simulink model "EHP_test"  (Simulink 7.4)
settings: Solver=FixedStepDiscrete  StartTime=0.0  StopTime=inf  FixedStep=0.01  RelTol=1e-3
undefined symbols (not defined in the file): EHPc_BatIsoTestCmd, EHPc_r_ClcnRo, EHPc_r_IsoDiag_limit, EHPc_r_IsoDiagInitVal, EHPc_r_IsoDiagWarn_limit
libraries: simulink x5
settings Model: Creator=zhaoxiangri  LastModifiedBy=sunsijun

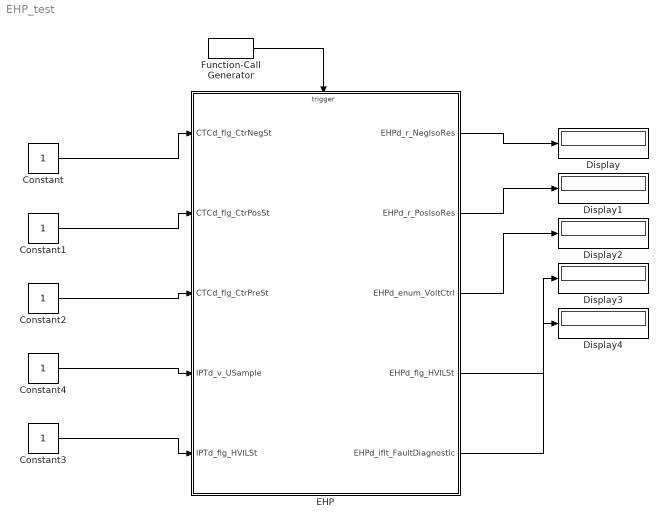
== system EHP_test ==
  Constant{,1..3} (4 alike) : Constant  OutDataTypeMode=boolean  OutDataType=fixdt(1, 16)  OutScaling=2^0  OutDataTypeStr=boolean
  Constant4 : Constant  OutDataTypeMode=single  OutDataType=fixdt(1, 16)  OutScaling=2^0  OutDataTypeStr=single
  Display{,1..4} (5 alike) : Display
  EHP : Subsystem  TreatAsAtomicUnit=on
  Function-Call Generator : simulink/Ports & Subsystems/Function-Call Generator  sample_time=1  numberOfIterations=1
  wires:
  Function-Call Generator/1 -> EHP/Trigger
  Constant/1 -> EHP/1(CTCd_flg_CtrNegSt)
  Constant1/1 -> EHP/2(CTCd_flg_CtrPosSt)
  Constant2/1 -> EHP/3(CTCd_flg_CtrPreSt)
  Constant3/1 -> EHP/5(IPTd_flg_HVILSt)
  Constant4/1 -> EHP/4(IPTd_v_USample)
  EHP/1(EHPd_r_NegIsoRes) -> Display/1
  EHP/2(EHPd_r_PosIsoRes) -> Display1/1
  EHP/3(EHPd_enum_VoltCtrl) -> Display2/1
  EHP/4(EHPd_flg_HVILSt) -> Display3/1
  EHP/5(EHPd_iflt_FaultDiagnostic) -> Display4/1

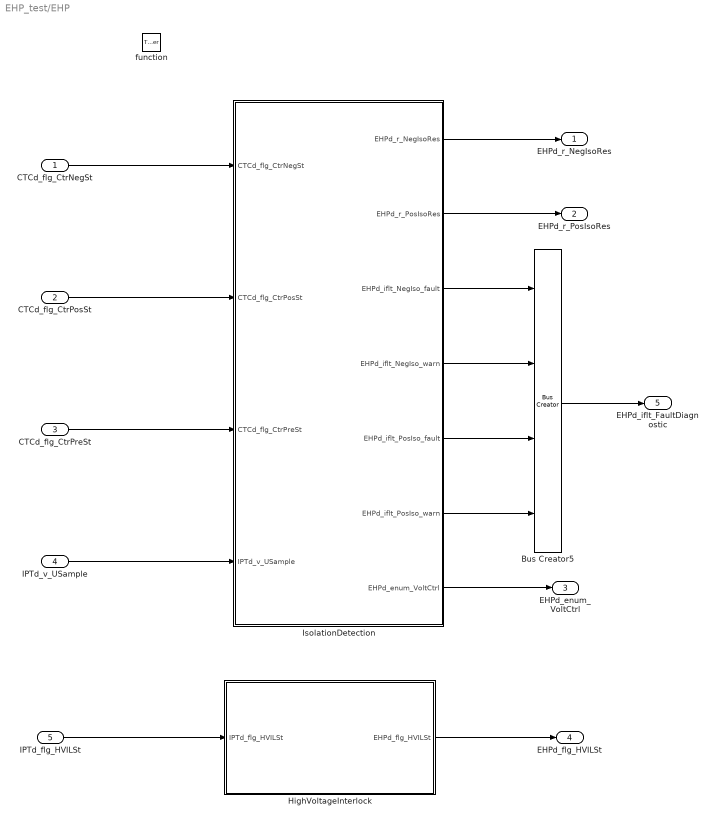
== system EHP_test/EHP ==
  CTCd_flg_CtrNegSt : Inport  OutDataType=fixdt(1, 16)  OutScaling=2^0
  CTCd_flg_CtrPosSt : Inport  Port=2  OutDataType=fixdt(1, 16)  OutScaling=2^0
  CTCd_flg_CtrPreSt : Inport  Port=3  OutDataType=fixdt(1, 16)  OutScaling=2^0
  IPTd_v_USample : Inport  Port=4  OutDataType=fixdt(1, 16)  OutScaling=2^0
  IPTd_flg_HVILSt : Inport  Port=5  OutDataType=fixdt(1, 16)  OutScaling=2^0
  function : TriggerPort  TriggerType=function-call
  Bus Creator5 : BusCreator
  HighVoltageInterlock : Subsystem  RTWFcnName=HighVoltageInterlock
      settings: RTWSystemCode=Function  RTWFcnNameOpts=User specified  RTWFileNameOpts=Use function name
  IsolationDetection : Subsystem  Description=|
      | $Author:Yan LiJuan$
      | $Date:2015/03/26$  
      | $Revision:1.0$
  EHPd_r_NegIsoRes : Outport  OutDataType=fixdt(1, 16)  OutScaling=2^0
  EHPd_r_PosIsoRes : Outport  Port=2  OutDataType=fixdt(1, 16)  OutScaling=2^0
  EHPd_enum_VoltCtrl : Outport  Port=3  OutDataType=fixdt(1, 16)  OutScaling=2^0
  EHPd_flg_HVILSt : Outport  Port=4  OutDataType=fixdt(1, 16)  OutScaling=2^0
  EHPd_iflt_FaultDiagnostic : Outport  Port=5  OutDataType=fixdt(1, 16)  OutScaling=2^0
  wires:
  IsolationDetection/7(EHPd_enum_VoltCtrl) -> EHPd_enum_VoltCtrl/1
  IsolationDetection/2(EHPd_r_PosIsoRes) -> EHPd_r_PosIsoRes/1
  IsolationDetection/1(EHPd_r_NegIsoRes) -> EHPd_r_NegIsoRes/1
  IPTd_flg_HVILSt/1 -> HighVoltageInterlock/1(IPTd_flg_HVILSt)
  HighVoltageInterlock/1(EHPd_flg_HVILSt) -> EHPd_flg_HVILSt/1
  IPTd_v_USample/1 -> IsolationDetection/4(IPTd_v_USample)
  CTCd_flg_CtrPreSt/1 -> IsolationDetection/3(CTCd_flg_CtrPreSt)
  CTCd_flg_CtrPosSt/1 -> IsolationDetection/2(CTCd_flg_CtrPosSt)
  CTCd_flg_CtrNegSt/1 -> IsolationDetection/1(CTCd_flg_CtrNegSt)
  IsolationDetection/3(EHPd_iflt_NegIso_fault) -> Bus Creator5/1
  IsolationDetection/4(EHPd_iflt_NegIso_warn) -> Bus Creator5/2
  IsolationDetection/5(EHPd_iflt_PosIso_fault) -> Bus Creator5/3
  IsolationDetection/6(EHPd_iflt_PosIso_warn) -> Bus Creator5/4
  Bus Creator5/1 -> EHPd_iflt_FaultDiagnostic/1

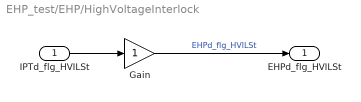
== system EHP_test/EHP/HighVoltageInterlock ==
  IPTd_flg_HVILSt : Inport  OutDataType=fixdt(1, 16)  OutScaling=2^0
  Gain : Gain  ParameterDataType=fixdt(1, 16)  ParameterScaling=2^0  OutDataType=fixdt(1, 16)  OutScaling=2^0
  EHPd_flg_HVILSt : Outport  OutDataType=fixdt(1, 16)  OutScaling=2^0
  wires:
  IPTd_flg_HVILSt/1 -> Gain/1
  Gain/1 -> EHPd_flg_HVILSt/1  "EHPd_flg_HVILSt"

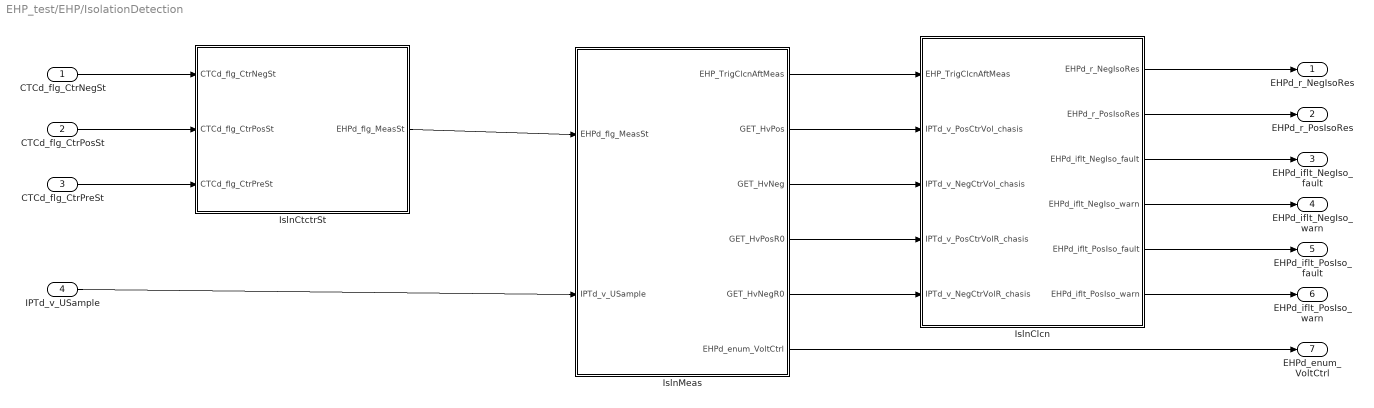
== system EHP_test/EHP/IsolationDetection ==
  CTCd_flg_CtrNegSt : Inport  OutDataType=fixdt(1, 16)  OutScaling=2^0
  CTCd_flg_CtrPosSt : Inport  Port=2  OutDataType=fixdt(1, 16)  OutScaling=2^0
  CTCd_flg_CtrPreSt : Inport  Port=3  OutDataType=fixdt(1, 16)  OutScaling=2^0
  IPTd_v_USample : Inport  Port=4  OutDataType=fixdt(1, 16)  OutScaling=2^0
  IslnClcn : Subsystem  Description=|
      | $Author:Yan LiJuan$
      | $Date:2015/03/26$  
      | $Revision:1.0$
  IslnCtctrSt : Subsystem  Description=|
      | $Author:Yan LiJuan$
      | $Date:2015/03/26$  
      | $Revision:1.0$
  IslnMeas : Subsystem  Description=|
      | $Author:Yan LiJuan$
      | $Date:2015/03/26$  
      | $Revision:1.0$
  EHPd_r_NegIsoRes : Outport  OutDataType=fixdt(1, 16)  OutScaling=2^0
  EHPd_r_PosIsoRes : Outport  Port=2  OutDataType=fixdt(1, 16)  OutScaling=2^0
  EHPd_iflt_NegIso_fault : Outport  Port=3  OutDataType=fixdt(1, 16)  OutScaling=2^0
  EHPd_iflt_NegIso_warn : Outport  Port=4  OutDataType=fixdt(1, 16)  OutScaling=2^0
  EHPd_iflt_PosIso_fault : Outport  Port=5  OutDataType=fixdt(1, 16)  OutScaling=2^0
  EHPd_iflt_PosIso_warn : Outport  Port=6  OutDataType=fixdt(1, 16)  OutScaling=2^0
  EHPd_enum_VoltCtrl : Outport  Port=7  OutDataType=fixdt(1, 16)  OutScaling=2^0
  wires:
  IslnMeas/6(EHPd_enum_VoltCtrl) -> EHPd_enum_VoltCtrl/1
  IslnClcn/6(EHPd_iflt_PosIso_warn) -> EHPd_iflt_PosIso_warn/1
  IslnClcn/5(EHPd_iflt_PosIso_fault) -> EHPd_iflt_PosIso_fault/1
  IslnClcn/4(EHPd_iflt_NegIso_warn) -> EHPd_iflt_NegIso_warn/1
  IslnClcn/3(EHPd_iflt_NegIso_fault) -> EHPd_iflt_NegIso_fault/1
  IslnClcn/2(EHPd_r_PosIsoRes) -> EHPd_r_PosIsoRes/1
  IslnClcn/1(EHPd_r_NegIsoRes) -> EHPd_r_NegIsoRes/1
  IslnMeas/4(GET_HvPosR0) -> IslnClcn/4(IPTd_v_PosCtrVolR_chasis)
  IslnMeas/1(EHP_TrigClcnAftMeas) -> IslnClcn/1(EHP_TrigClcnAftMeas)
  CTCd_flg_CtrPreSt/1 -> IslnCtctrSt/3(CTCd_flg_CtrPreSt)
  CTCd_flg_CtrPosSt/1 -> IslnCtctrSt/2(CTCd_flg_CtrPosSt)
  CTCd_flg_CtrNegSt/1 -> IslnCtctrSt/1(CTCd_flg_CtrNegSt)
  IslnMeas/5(GET_HvNegR0) -> IslnClcn/5(IPTd_v_NegCtrVolR_chasis)
  IPTd_v_USample/1 -> IslnMeas/2(IPTd_v_USample)
  IslnMeas/3(GET_HvNeg) -> IslnClcn/3(IPTd_v_NegCtrVol_chasis)
  IslnCtctrSt/1(EHPd_flg_MeasSt) -> IslnMeas/1(EHPd_flg_MeasSt)
  IslnMeas/2(GET_HvPos) -> IslnClcn/2(IPTd_v_PosCtrVol_chasis)

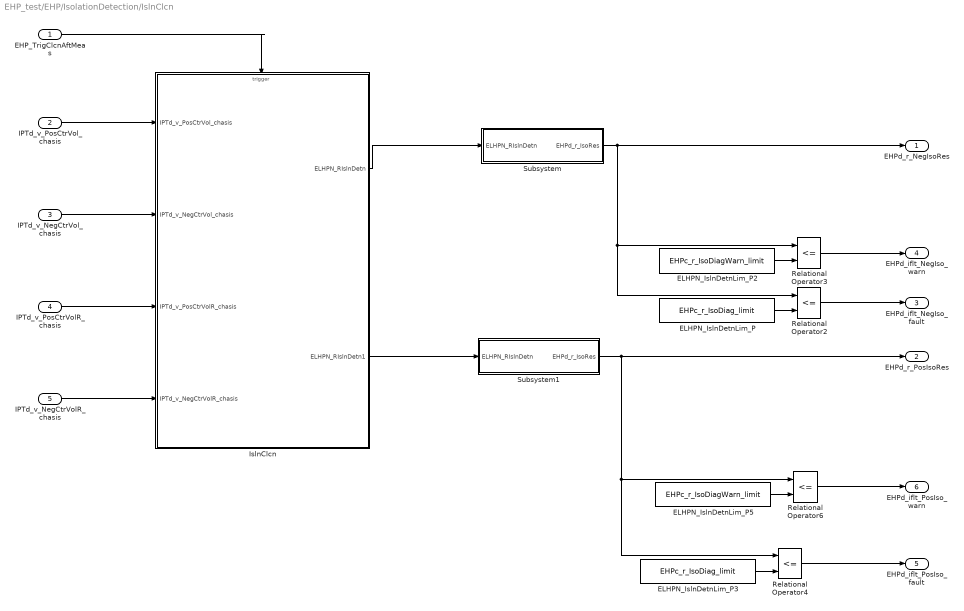
== system EHP_test/EHP/IsolationDetection/IslnClcn ==
  EHP_TrigClcnAftMeas : Inport  OutDataType=fixdt(1, 16)  OutScaling=2^0
  IPTd_v_PosCtrVol_chasis : Inport  Port=2  OutDataType=fixdt(1, 16)  OutScaling=2^0
  IPTd_v_NegCtrVol_chasis : Inport  Port=3  OutDataType=fixdt(1, 16)  OutScaling=2^0
  IPTd_v_PosCtrVolR_chasis : Inport  Port=4  OutDataType=fixdt(1, 16)  OutScaling=2^0
  IPTd_v_NegCtrVolR_chasis : Inport  Port=5  OutDataType=fixdt(1, 16)  OutScaling=2^0
  ELHPN_IslnDetnLim_P : Constant  Value=EHPc_r_IsoDiag_limit  OutDataType=fixdt(1, 16)  OutScaling=2^0
  ELHPN_IslnDetnLim_P2 : Constant  Value=EHPc_r_IsoDiagWarn_limit  OutDataType=fixdt(1, 16)  OutScaling=2^0
  ELHPN_IslnDetnLim_P3 : Constant  Value=EHPc_r_IsoDiag_limit  OutDataType=fixdt(1, 16)  OutScaling=2^0
  ELHPN_IslnDetnLim_P5 : Constant  Value=EHPc_r_IsoDiagWarn_limit  OutDataType=fixdt(1, 16)  OutScaling=2^0
  IslnClcn : Subsystem  Description=|
      | $Author:Yan LiJuan$
      | $Date:2015/03/26$  
      | $Revision:1.0$
  Relational Operator{2..4,6} (4 alike) : RelationalOperator  Operator=<=  LogicOutDataTypeMode=boolean  LogicDataType=fixdt(0, 8)  OutDataTypeStr=boolean
  Subsystem : Subsystem
  Subsystem1 : Subsystem
  EHPd_r_NegIsoRes : Outport  OutDataType=fixdt(1, 16)  OutScaling=2^0
  EHPd_r_PosIsoRes : Outport  Port=2  OutDataType=fixdt(1, 16)  OutScaling=2^0
  EHPd_iflt_NegIso_fault : Outport  Port=3  OutDataType=fixdt(1, 16)  OutScaling=2^0
  EHPd_iflt_NegIso_warn : Outport  Port=4  OutDataType=fixdt(1, 16)  OutScaling=2^0
  EHPd_iflt_PosIso_fault : Outport  Port=5  OutDataType=fixdt(1, 16)  OutScaling=2^0
  EHPd_iflt_PosIso_warn : Outport  Port=6  OutDataType=fixdt(1, 16)  OutScaling=2^0
  wires:
  Relational Operator6/1 -> EHPd_iflt_PosIso_warn/1
  ELHPN_IslnDetnLim_P5/1 -> Relational Operator6/2
  Relational Operator3/1 -> EHPd_iflt_NegIso_warn/1
  Relational Operator4/1 -> EHPd_iflt_PosIso_fault/1
  ELHPN_IslnDetnLim_P3/1 -> Relational Operator4/2
  ELHPN_IslnDetnLim_P2/1 -> Relational Operator3/2
  IslnClcn/2(ELHPN_RIslnDetn1) -> Subsystem1/1(ELHPN_RIslnDetn)
  Subsystem1/1(EHPd_r_IsoRes) -> Relational Operator4/1, Relational Operator6/1, EHPd_r_PosIsoRes/1
  IPTd_v_NegCtrVolR_chasis/1 -> IslnClcn/4(IPTd_v_NegCtrVolR_chasis)
  IPTd_v_PosCtrVolR_chasis/1 -> IslnClcn/3(IPTd_v_PosCtrVolR_chasis)
  IPTd_v_NegCtrVol_chasis/1 -> IslnClcn/2(IPTd_v_NegCtrVol_chasis)
  IPTd_v_PosCtrVol_chasis/1 -> IslnClcn/1(IPTd_v_PosCtrVol_chasis)
  EHP_TrigClcnAftMeas/1 -> IslnClcn/Trigger
  IslnClcn/1(ELHPN_RIslnDetn) -> Subsystem/1(ELHPN_RIslnDetn)
  Relational Operator2/1 -> EHPd_iflt_NegIso_fault/1
  Subsystem/1(EHPd_r_IsoRes) -> Relational Operator2/1, Relational Operator3/1, EHPd_r_NegIsoRes/1
  ELHPN_IslnDetnLim_P/1 -> Relational Operator2/2

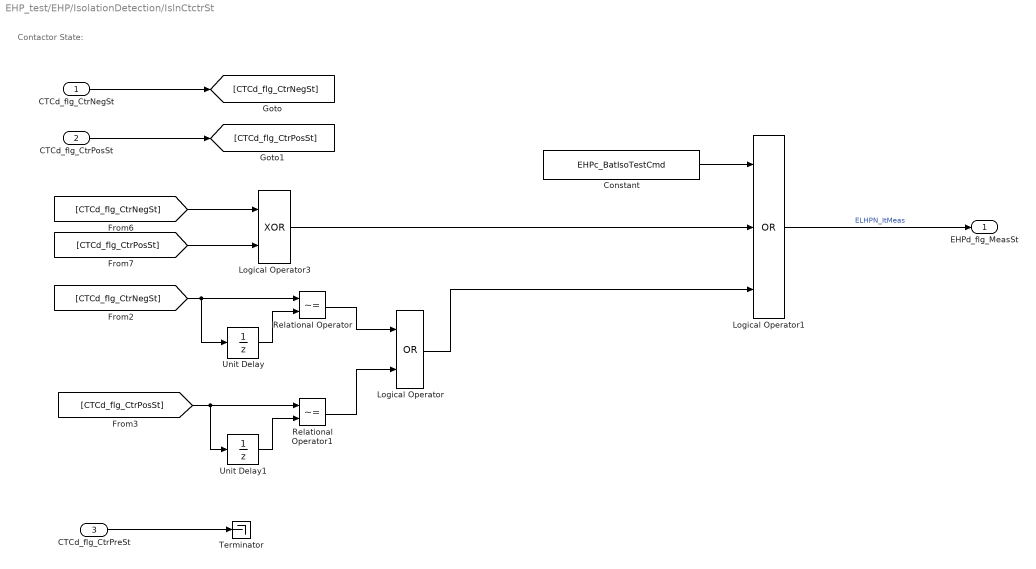
== system EHP_test/EHP/IsolationDetection/IslnCtctrSt ==
  note: Contactor State:
  CTCd_flg_CtrNegSt : Inport  OutDataType=fixdt(1, 16)  OutScaling=2^0
  CTCd_flg_CtrPosSt : Inport  Port=2  OutDataType=fixdt(1, 16)  OutScaling=2^0
  CTCd_flg_CtrPreSt : Inport  Port=3  OutDataType=fixdt(1, 16)  OutScaling=2^0
  Constant : Constant  Value=EHPc_BatIsoTestCmd  OutDataTypeMode=boolean  OutDataType=fixdt(1, 16)  OutScaling=2^0  OutDataTypeStr=boolean
  Logical Operator : Logic  Operator=OR  AllPortsSameDT=off  OutDataTypeMode=boolean  LogicDataType=fixdt(0, 8)  OutDataTypeStr=boolean
  Logical Operator1 : Logic  Operator=OR  Inputs=3  AllPortsSameDT=off  OutDataTypeMode=boolean  LogicDataType=fixdt(0, 8)  OutDataTypeStr=boolean
  Logical Operator3 : Logic  Operator=XOR  AllPortsSameDT=off  OutDataTypeMode=boolean  LogicDataType=fixdt(0, 8)  OutDataTypeStr=boolean
  Relational Operator : RelationalOperator  Operator=~=  LogicOutDataTypeMode=boolean  LogicDataType=fixdt(0, 8)  OutDataTypeStr=boolean
  Relational Operator1 : RelationalOperator  Operator=~=  LogicOutDataTypeMode=boolean  LogicDataType=fixdt(0, 8)  OutDataTypeStr=boolean
  Terminator : Terminator
  Unit Delay : UnitDelay  SampleTime=-1
  Unit Delay1 : UnitDelay  SampleTime=-1
  EHPd_flg_MeasSt : Outport  OutDataType=fixdt(1, 16)  OutScaling=2^0
  wires:
  Constant/1 -> Logical Operator1/1
  Logical Operator1/1 -> EHPd_flg_MeasSt/1  "ELHPN_ItMeas"
  CTCd_flg_CtrPreSt/1 -> Terminator/1
  Logical Operator3/1 -> Logical Operator1/2
  Logical Operator/1 -> Logical Operator1/3
  [CTCd_flg_CtrPosSt] -> Logical Operator3/2
  [CTCd_flg_CtrNegSt] -> Logical Operator3/1
  Relational Operator1/1 -> Logical Operator/2
  Relational Operator/1 -> Logical Operator/1
  Unit Delay1/1 -> Relational Operator1/2
  [CTCd_flg_CtrPosSt] -> Unit Delay1/1, Relational Operator1/1
  Unit Delay/1 -> Relational Operator/2
  [CTCd_flg_CtrNegSt] -> Unit Delay/1, Relational Operator/1
  CTCd_flg_CtrPosSt/1 -> [CTCd_flg_CtrPosSt]
  CTCd_flg_CtrNegSt/1 -> [CTCd_flg_CtrNegSt]

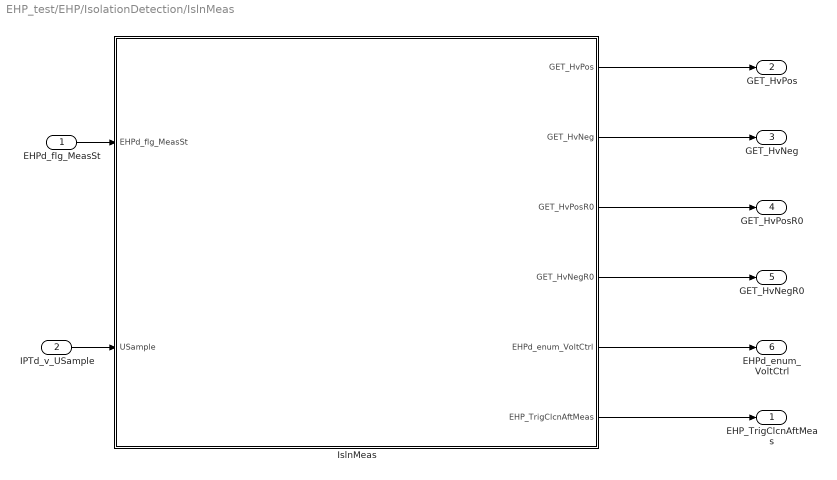
== system EHP_test/EHP/IsolationDetection/IslnMeas ==
  EHPd_flg_MeasSt : Inport  DataType=boolean  OutDataType=fixdt(1, 16)  OutScaling=2^0  OutDataTypeStr=boolean
  IPTd_v_USample : Inport  Port=2  OutDataType=fixdt(1, 16)  OutScaling=2^0
  IslnMeas : Stateflow chart  Description=|
      | $Author:Yan LiJuan$
      | $Date:2015/03/26$  
      | $Revision:1.0$
  EHP_TrigClcnAftMeas : Outport  OutDataType=fixdt(1, 16)  OutScaling=2^0
  GET_HvPos : Outport  Port=2  OutDataType=fixdt(1, 16)  OutScaling=2^0
  GET_HvNeg : Outport  Port=3  OutDataType=fixdt(1, 16)  OutScaling=2^0
  GET_HvPosR0 : Outport  Port=4  OutDataType=fixdt(1, 16)  OutScaling=2^0
  GET_HvNegR0 : Outport  Port=5  OutDataType=fixdt(1, 16)  OutScaling=2^0
  EHPd_enum_VoltCtrl : Outport  Port=6  OutDataType=fixdt(1, 16)  OutScaling=2^0
  wires:
  IslnMeas/5(EHPd_enum_VoltCtrl) -> EHPd_enum_VoltCtrl/1
  EHPd_flg_MeasSt/1 -> IslnMeas/1(EHPd_flg_MeasSt)
  IslnMeas/6(EHP_TrigClcnAftMeas) -> EHP_TrigClcnAftMeas/1
  IslnMeas/4(GET_HvNegR0) -> GET_HvNegR0/1
  IslnMeas/3(GET_HvPosR0) -> GET_HvPosR0/1
  IslnMeas/2(GET_HvNeg) -> GET_HvNeg/1
  IslnMeas/1(GET_HvPos) -> GET_HvPos/1
  IPTd_v_USample/1 -> IslnMeas/2(USample)

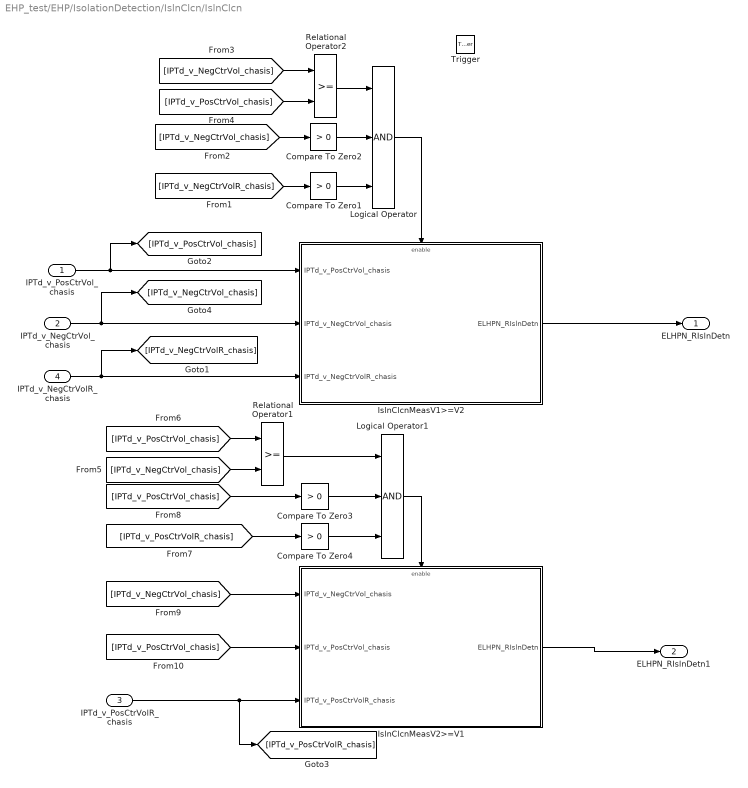
== system EHP_test/EHP/IsolationDetection/IslnClcn/IslnClcn ==
  IPTd_v_PosCtrVol_chasis : Inport  OutDataType=fixdt(1, 16)  OutScaling=2^0
  IPTd_v_NegCtrVol_chasis : Inport  Port=2  OutDataType=fixdt(1, 16)  OutScaling=2^0
  IPTd_v_PosCtrVolR_chasis : Inport  Port=3  OutDataType=fixdt(1, 16)  OutScaling=2^0
  IPTd_v_NegCtrVolR_chasis : Inport  Port=4  OutDataType=fixdt(1, 16)  OutScaling=2^0
  Trigger : TriggerPort
  Compare To Zero{1..4} (4 alike) : simulink/Logic and Bit Operations/Compare To Zero  SystemSampleTime=-1  relop=>  LogicOutDataTypeMode=uint8
  IslnClcnMeasV1>=V2 : Subsystem  TreatAsAtomicUnit=on
  IslnClcnMeasV2>=V1 : Subsystem  TreatAsAtomicUnit=on
  Logical Operator : Logic  Inputs=3  AllPortsSameDT=off  OutDataTypeMode=boolean  LogicDataType=fixdt(0, 8)  OutDataTypeStr=boolean
  Logical Operator1 : Logic  Inputs=3  AllPortsSameDT=off  OutDataTypeMode=boolean  LogicDataType=fixdt(0, 8)  OutDataTypeStr=boolean
  Relational Operator1 : RelationalOperator  LogicOutDataTypeMode=boolean  LogicDataType=fixdt(0, 8)  OutDataTypeStr=boolean
  Relational Operator2 : RelationalOperator  LogicOutDataTypeMode=boolean  LogicDataType=fixdt(0, 8)  OutDataTypeStr=boolean
  ELHPN_RIslnDetn : Outport  OutDataType=fixdt(1, 16)  OutScaling=2^0
  ELHPN_RIslnDetn1 : Outport  Port=2  OutDataType=fixdt(1, 16)  OutScaling=2^0
  wires:
  Compare To Zero4/1 -> Logical Operator1/3
  Compare To Zero3/1 -> Logical Operator1/2
  Relational Operator1/1 -> Logical Operator1/1
  [IPTd_v_NegCtrVol_chasis] -> Relational Operator1/2
  [IPTd_v_PosCtrVol_chasis] -> Relational Operator1/1
  Compare To Zero1/1 -> Logical Operator/3
  Compare To Zero2/1 -> Logical Operator/2
  Relational Operator2/1 -> Logical Operator/1
  [IPTd_v_PosCtrVol_chasis] -> Relational Operator2/2
  [IPTd_v_NegCtrVol_chasis] -> Relational Operator2/1
  Logical Operator1/1 -> IslnClcnMeasV2>=V1/Enable
  [IPTd_v_PosCtrVolR_chasis] -> Compare To Zero4/1
  [IPTd_v_PosCtrVol_chasis] -> Compare To Zero3/1
  IslnClcnMeasV2>=V1/1(ELHPN_RIslnDetn) -> ELHPN_RIslnDetn1/1
  IslnClcnMeasV1>=V2/1(ELHPN_RIslnDetn) -> ELHPN_RIslnDetn/1
  [IPTd_v_NegCtrVolR_chasis] -> Compare To Zero1/1
  [IPTd_v_NegCtrVol_chasis] -> Compare To Zero2/1
  Logical Operator/1 -> IslnClcnMeasV1>=V2/Enable
  IPTd_v_PosCtrVolR_chasis/1 -> [IPTd_v_PosCtrVolR_chasis], IslnClcnMeasV2>=V1/3(IPTd_v_PosCtrVolR_chasis)
  [IPTd_v_PosCtrVol_chasis] -> IslnClcnMeasV2>=V1/2(IPTd_v_PosCtrVol_chasis)
  [IPTd_v_NegCtrVol_chasis] -> IslnClcnMeasV2>=V1/1(IPTd_v_NegCtrVol_chasis)
  IPTd_v_NegCtrVolR_chasis/1 -> [IPTd_v_NegCtrVolR_chasis], IslnClcnMeasV1>=V2/3(IPTd_v_NegCtrVolR_chasis)
  IPTd_v_PosCtrVol_chasis/1 -> IslnClcnMeasV1>=V2/1(IPTd_v_PosCtrVol_chasis), [IPTd_v_PosCtrVol_chasis]
  IPTd_v_NegCtrVol_chasis/1 -> [IPTd_v_NegCtrVol_chasis], IslnClcnMeasV1>=V2/2(IPTd_v_NegCtrVol_chasis)

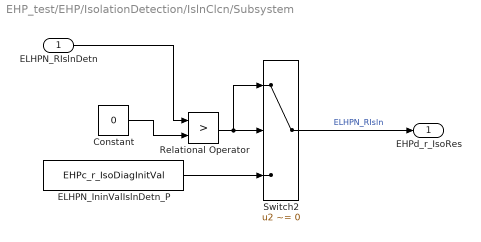
== system EHP_test/EHP/IsolationDetection/IslnClcn/Subsystem ==
  ELHPN_RIslnDetn : Inport  OutDataType=fixdt(1, 16)  OutScaling=2^0
  Constant : Constant  Value=0  OutDataType=fixdt(1, 16)  OutScaling=2^0
  ELHPN_IninValIslnDetn_P : Constant  Value=EHPc_r_IsoDiagInitVal  OutDataType=fixdt(1, 16)  OutScaling=2^0
  Relational Operator : RelationalOperator  Operator=>  LogicOutDataTypeMode=boolean  LogicDataType=fixdt(0, 8)  OutDataTypeStr=boolean
  Switch2 : Switch  Criteria=u2 ~= 0  OutDataType=fixdt(1, 16)  OutScaling=2^0
  EHPd_r_IsoRes : Outport  OutDataType=fixdt(1, 16)  OutScaling=2^0
  wires:
  ELHPN_IninValIslnDetn_P/1 -> Switch2/3
  Relational Operator/1 -> Switch2/2, Switch2/1
  Constant/1 -> Relational Operator/2
  ELHPN_RIslnDetn/1 -> Relational Operator/1
  Switch2/1 -> EHPd_r_IsoRes/1  "ELHPN_RIsln"

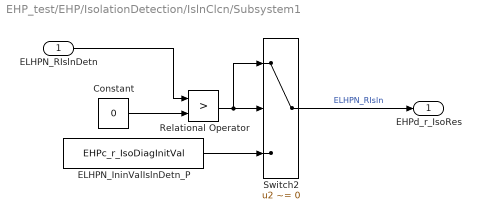
== system EHP_test/EHP/IsolationDetection/IslnClcn/Subsystem1 ==
  ELHPN_RIslnDetn : Inport  OutDataType=fixdt(1, 16)  OutScaling=2^0
  Constant : Constant  Value=0  OutDataType=fixdt(1, 16)  OutScaling=2^0
  ELHPN_IninValIslnDetn_P : Constant  Value=EHPc_r_IsoDiagInitVal  OutDataType=fixdt(1, 16)  OutScaling=2^0
  Relational Operator : RelationalOperator  Operator=>  LogicOutDataTypeMode=boolean  LogicDataType=fixdt(0, 8)  OutDataTypeStr=boolean
  Switch2 : Switch  Criteria=u2 ~= 0  OutDataType=fixdt(1, 16)  OutScaling=2^0
  EHPd_r_IsoRes : Outport  OutDataType=fixdt(1, 16)  OutScaling=2^0
  wires:
  ELHPN_IninValIslnDetn_P/1 -> Switch2/3
  Relational Operator/1 -> Switch2/2, Switch2/1
  Constant/1 -> Relational Operator/2
  ELHPN_RIslnDetn/1 -> Relational Operator/1
  Switch2/1 -> EHPd_r_IsoRes/1  "ELHPN_RIsln"

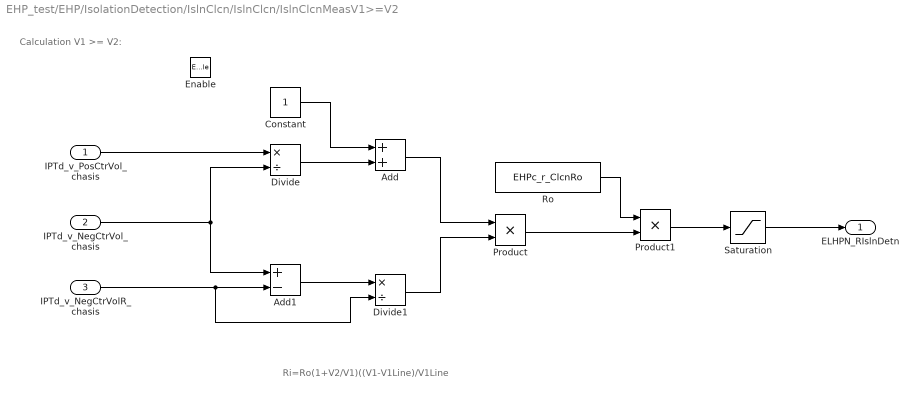
== system EHP_test/EHP/IsolationDetection/IslnClcn/IslnClcn/IslnClcnMeasV1>=V2 ==
  note: Calculation V1 >= V2:
  note: Ri=Ro(1+V2/V1)((V1-V1Line)/V1Line
  IPTd_v_PosCtrVol_chasis : Inport  OutDataType=fixdt(1, 16)  OutScaling=2^0
  IPTd_v_NegCtrVol_chasis : Inport  Port=2  OutDataType=fixdt(1, 16)  OutScaling=2^0
  IPTd_v_NegCtrVolR_chasis : Inport  Port=3  OutDataType=fixdt(1, 16)  OutScaling=2^0
  Enable : EnablePort
  Add : Sum  OutDataType=fixdt(1, 16)  OutScaling=2^-10  SaturateOnIntegerOverflow=on
  Add1 : Sum  Inputs=+-  OutDataType=fixdt(1, 16)  OutScaling=2^-10  SaturateOnIntegerOverflow=on
  Constant : Constant  OutDataType=fixdt(1, 16)  OutScaling=2^0
  Divide : Product  Inputs=*/  OutDataType=fixdt(1, 16)  OutScaling=2^-10  SaturateOnIntegerOverflow=on
  Divide1 : Product  Inputs=*/  OutDataType=fixdt(1, 16)  OutScaling=2^-10  SaturateOnIntegerOverflow=on
  Product : Product  OutDataType=fixdt(1, 16)  OutScaling=2^0  SaturateOnIntegerOverflow=on  RndMeth=Zero
  Product1 : Product  OutDataType=fixdt(1, 16)  OutScaling=2^0  SaturateOnIntegerOverflow=on  RndMeth=Zero
  Ro : Constant  Value=EHPc_r_ClcnRo  OutDataType=fixdt(1, 16)  OutScaling=2^0
  Saturation : Saturate  UpperLimit=10000000  LowerLimit=1  OutDataType=fixdt(1, 16)  OutScaling=2^0
  ELHPN_RIslnDetn : Outport  OutDataType=fixdt(1, 16)  OutScaling=2^0
  wires:
  Ro/1 -> Product1/1
  Product1/1 -> Saturation/1
  Product/1 -> Product1/2
  Divide1/1 -> Product/2
  Add/1 -> Product/1
  Add1/1 -> Divide1/1
  IPTd_v_NegCtrVolR_chasis/1 -> Divide1/2, Add1/2
  Constant/1 -> Add/1
  Divide/1 -> Add/2
  IPTd_v_NegCtrVol_chasis/1 -> Add1/1, Divide/2
  IPTd_v_PosCtrVol_chasis/1 -> Divide/1
  Saturation/1 -> ELHPN_RIslnDetn/1

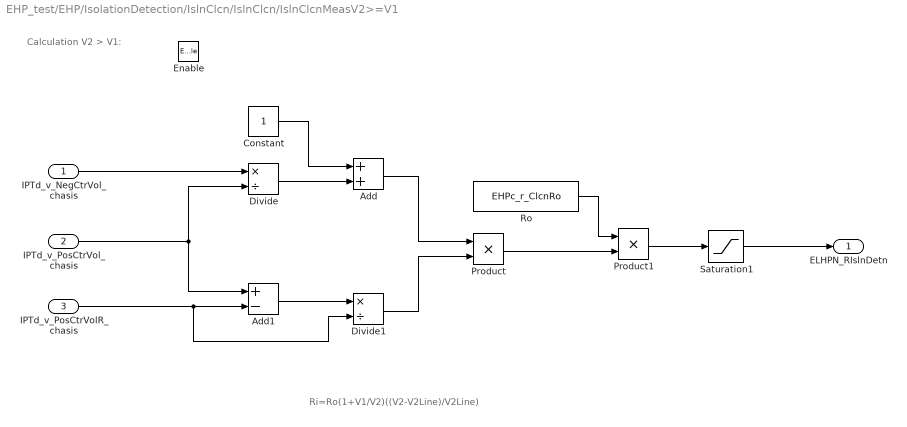
== system EHP_test/EHP/IsolationDetection/IslnClcn/IslnClcn/IslnClcnMeasV2>=V1 ==
  note: Calculation V2 > V1:
  note: Ri=Ro(1+V1/V2)((V2-V2Line)/V2Line)
  IPTd_v_NegCtrVol_chasis : Inport  OutDataType=fixdt(1, 16)  OutScaling=2^0
  IPTd_v_PosCtrVol_chasis : Inport  Port=2  OutDataType=fixdt(1, 16)  OutScaling=2^0
  IPTd_v_PosCtrVolR_chasis : Inport  Port=3  OutDataType=fixdt(1, 16)  OutScaling=2^0
  Enable : EnablePort
  Add : Sum  OutDataType=fixdt(1, 16)  OutScaling=2^-10
  Add1 : Sum  Inputs=+-  OutDataType=fixdt(1, 16)  OutScaling=2^-10
  Constant : Constant  OutDataType=fixdt(1, 16)  OutScaling=2^0
  Divide : Product  Inputs=*/  OutDataType=fixdt(1, 16)  OutScaling=2^-10
  Divide1 : Product  Inputs=*/  OutDataType=fixdt(1, 16)  OutScaling=2^-10
  Product : Product  OutDataType=fixdt(1, 16)  OutScaling=2^0  RndMeth=Zero
  Product1 : Product  OutDataType=fixdt(1, 16)  OutScaling=2^0  RndMeth=Zero
  Ro : Constant  Value=EHPc_r_ClcnRo  OutDataType=fixdt(1, 16)  OutScaling=2^0
  Saturation1 : Saturate  UpperLimit=10000000  LowerLimit=1  OutDataType=fixdt(1, 16)  OutScaling=2^0
  ELHPN_RIslnDetn : Outport  OutDataType=fixdt(1, 16)  OutScaling=2^0
  wires:
  Ro/1 -> Product1/1
  Product1/1 -> Saturation1/1
  Product/1 -> Product1/2
  Divide1/1 -> Product/2
  Add/1 -> Product/1
  Add1/1 -> Divide1/1
  IPTd_v_PosCtrVolR_chasis/1 -> Divide1/2, Add1/2
  Constant/1 -> Add/1
  Divide/1 -> Add/2
  IPTd_v_PosCtrVol_chasis/1 -> Add1/1, Divide/2
  IPTd_v_NegCtrVol_chasis/1 -> Divide/1
  Saturation1/1 -> ELHPN_RIslnDetn/1

== stateflow chart EHP/IsolationDetection/IslnMeas/IslnMeas ==
  settings: description=|
      | $Author:Yan LiJuan$
      | $Date:2015/03/26$
      | $Revision:1.0$
  state Meas
    state State0
      EHPd_enum_StMeasIso=0;
    state UMeas
      state State1
        EHPd_enum_StMeasIso=1;
        du:EHPd_tm_MeasIso = EHPd_tm_MeasIso+0.1;
      state State2
        EHPd_enum_StMeasIso=2;
        du:EHPd_tm_MeasIso = EHPd_tm_MeasIso+0.1;
      state State4
        EHPd_enum_StMeasIso=4;
        du:EHPd_tm_MeasIso= EHPd_tm_MeasIso+0.1;
      state State3
        EHPd_enum_StMeasIso=3;
        du:EHPd_tm_MeasIso= EHPd_tm_MeasIso+0.1;
      state State5
        EHPd_enum_StMeasIso=5;
        du:EHPd_tm_MeasIso = EHPd_tm_MeasIso+0.1;
      state State6
        EHPd_enum_StMeasIso=6;
        du:EHPd_tm_MeasIso = EHPd_tm_MeasIso+0.1;
      state State7
        EHPd_enum_StMeasIso=7;
        du:EHPd_tm_MeasIso= EHPd_tm_MeasIso+0.1;
      state State8
        EHPd_enum_StMeasIso=8;
        du:EHPd_tm_MeasIso= EHPd_tm_MeasIso+0.1;
      (default) -> State1 : {EHPd_tm_MeasIso = 0;EHPd_enum_VoltCtrl = EHP_HvCtrl_St;}
      State1 -> State2 : [EHPd_tm_MeasIso >= EHPc_tm_MeasIso1_P]
          | {EHPd_tm_MeasIso = 0;EHPd_enum_VoltCtrl = EHP_HvPosCtrl_St;}
      State2 -> State3 : [EHPd_tm_MeasIso >= EHPc_tm_MeasIso2_P]
          | {EHPd_tm_MeasIso = 0;GET_HvPos=USample;EHPd_enum_VoltCtrl = EHP_HvCtrl_St;}
      State3 -> State4 : [EHPd_tm_MeasIso >= EHPc_tm_MeasIso3_P]
          | {EHPd_tm_MeasIso = 0;EHPd_enum_VoltCtrl = EHP_HvNegCtrl_St;}
      State4 -> State5 : [EHPd_tm_MeasIso >= EHPc_tm_MeasIso4_P]
          | {EHPd_tm_MeasIso = 0;GET_HvNeg=USample;EHPd_enum_VoltCtrl = EHP_HvCtrl_St;}
      State5 -> State6 : [EHPd_tm_MeasIso >= EHPc_tm_MeasIso5_P]
          | {EHPd_tm_MeasIso = 0;EHPd_enum_VoltCtrl = EHP_HvPosR0Ctrl_St;}
      State6 -> State7 : [EHPd_tm_MeasIso >= EHPc_tm_MeasIso6_P]
          | {EHPd_tm_MeasIso = 0;GET_HvPosR0=USample;EHPd_enum_VoltCtrl = EHP_HvCtrl_St;}
      State7 -> State8 : [EHPd_tm_MeasIso >= EHPc_tm_MeasIso7_P]
          | {EHPd_tm_MeasIso = 0;EHPd_enum_VoltCtrl = EHP_HvNegR0Ctrl_St;}
      State8 -> (junction 15) : [EHPd_tm_MeasIso >= EHPc_tm_MeasIso8_P]
          | {GET_HvNegR0=USample;EHPd_enum_VoltCtrl = EHP_HvCtrl_St;}
    (default) -> UMeas
    State0 -> UMeas : [EHPd_flg_MeasSt==0]
    UMeas -> State0 : [EHPd_flg_MeasSt==1]
  state Wait
    EHPd_enum_StMeasIso=7;
    du:
    EHPd_tm_Wait=EHPd_tm_Wait+0.1;
  (junction 15) -> Wait : {EHPd_tm_Wait=0;EHP_TrigClcnAftMeas;}
  (default) -> Meas
  Wait -> Meas : [EHPd_tm_Wait>=EHPc_tm_Wait_P]
  data: EHPd_tm_MeasIso local double; EHPc_tm_MeasIso1_P parameter double; EHPc_tm_MeasIso2_P parameter double; EHPc_tm_MeasIso3_P parameter double; EHPc_tm_MeasIso4_P parameter double; EHPc_tm_MeasIso5_P parameter double; EHPc_tm_MeasIso6_P parameter double; EHPc_tm_MeasIso7_P parameter double; EHPc_tm_MeasIso8_P parameter double; EHPd_flg_MeasSt input boolean; USample input double; GET_HvPos output double; GET_HvNeg output double; GET_HvPosR0 output double; GET_HvNegR0 output double; EHPd_enum_StMeasIso local double; EHPd_tm_Wait local double; EHPc_tm_Wait_P parameter double; EHPd_enum_VoltCtrl output double; EHP_HvCtrl_St parameter double; EHP_HvNegCtrl_St parameter double; EHP_HvNegR0Ctrl_St parameter double; EHP_HvPosCtrl_St parameter double; EHP_HvPosR0Ctrl_St parameter double
  events: EHP_TrigClcnAftMeas output EITHER_EDGE_EVENT
